simulink model "modelo_velocidade"  (R2023b)
settings: Solver=ode14x  StartTime=0.0  StopTime=4.5  FixedStep=0.01  RelTol=1e-3
values from neighbouring files (symbols this model uses):
  a = parametros (1)    [erro_velocidades_FINAL.m]
  b = parametros (2)    [erro_velocidades_FINAL.m]
  K = parametros (3)    [erro_velocidades_FINAL.m]
  PosReal = p(1:3000)    [Velocidades_FINAL.m]
  T = t(1:3000)    [Velocidades_FINAL.m]
  VDes = vDes(1:3000)    [Velocidades_FINAL.m]
libraries: eeGeneralControl x1
settings Model: Creator=alexa  LastModifiedBy=alexa

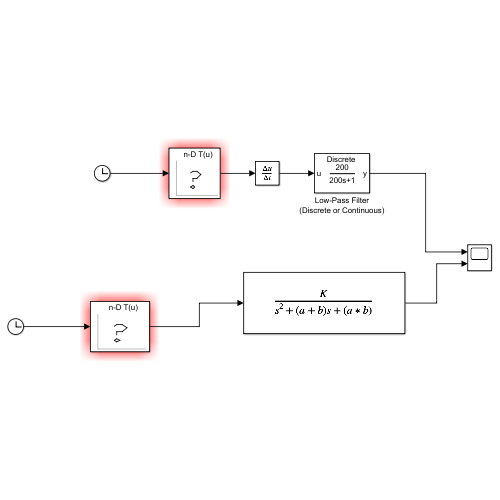
[thumbnail: Simulink's stored preview of the top-level diagram]
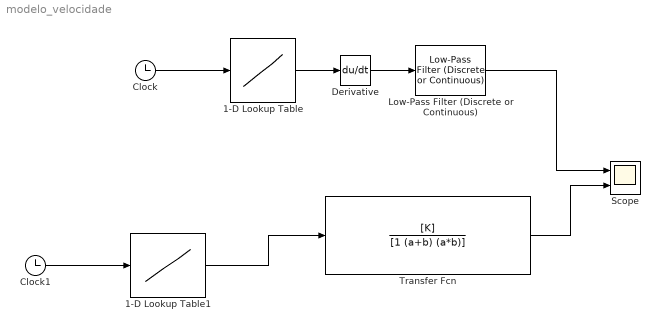
== system modelo_velocidade ==
  1-D Lookup Table : Lookup_n-D  NumberOfTableDimensions=1  BreakpointsForDimension1=T  Table=PosReal  InternalRulePriority=Speed  RndMeth=Simplest
  1-D Lookup Table1 : Lookup_n-D  NumberOfTableDimensions=1  BreakpointsForDimension1=T  Table=VDes  InternalRulePriority=Speed  RndMeth=Simplest
  Clock : Clock
  Clock1 : Clock
  Derivative : Derivative
  Low-Pass Filter (Discrete or Continuous) : eeGeneralControl/Low-Pass Filter (Discrete or Continuous)  K=200  T=200  B=inf  A=-inf  init_option=Inherited from block input  x0=0  Ts=-1
  Scope : Scope  NumInputPorts=2
  Transfer Fcn : TransferFcn  Numerator=[K]  Denominator=[1 (a+b) (a*b)]
  wires:
  Clock/1 -> 1-D Lookup Table/1
  Clock1/1 -> 1-D Lookup Table1/1
  1-D Lookup Table1/1 -> Transfer Fcn/1
  1-D Lookup Table/1 -> Derivative/1
  Derivative/1 -> Low-Pass Filter (Discrete or Continuous)/1
  Low-Pass Filter (Discrete or Continuous)/1 -> Scope/1
  Transfer Fcn/1 -> Scope/2
